simulink model "Test"  (R2018b)
settings: Solver=VariableStepAuto  StartTime=0.0  StopTime=3.0  RelTol=1e-3
libraries: dspvision x6, dspstat3 x5
settings Model: Creator=dell  LastModifiedBy=dell

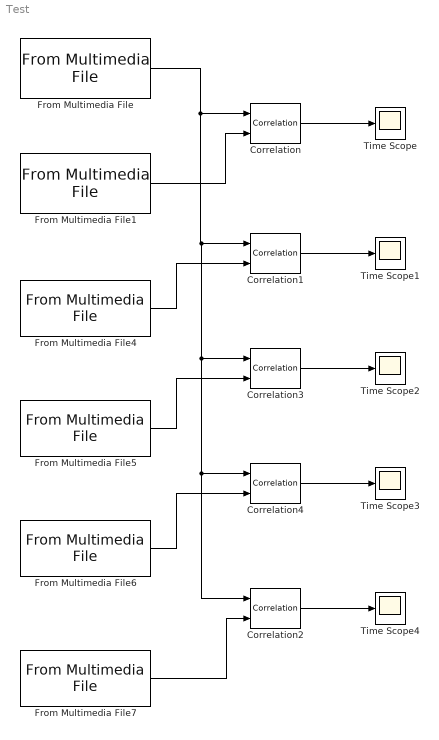
== system Test ==
  Correlation{,1..4} (5 alike) : dspstat3/Correlation  domain=Time  roundingMode=Floor  overflowMode=off  outputDataTypeStr=Inherit: Same as accumulator  outputMin=[]  outputMax=[]  outputLastDataTypeStr=Inherit: Same as accumulator
      settings: SourceProductName=DSP System Toolbox  SourceProductBaseCode=DS
  From Multimedia File : dspvision/From Multimedia File  inputFilename=C:\Users\dell\Desktop\Tone-Identification-master\test.wav  loop=on  numPlays=inf  outputStreams=Audio only  videoDataType=single  audioDataType=double  inheritSampleTime=on  userDefinedSampleTime=1/30  noAudioOutput=off  isIntensityVideo=off  fourcc=RGB  colorVideoFormat=Separate color signals  outputEOF=off  dataOrg=Column-major  audioFrameSize=10000  computeAudioFrameSize=off  outSamplingMode=Sample based
      settings: SourceProductBaseCode=VP
  From Multimedia File1 : dspvision/From Multimedia File  inputFilename=C:\Users\dell\Desktop\Tone-Identification-master\one.wav  loop=on  numPlays=inf  outputStreams=Audio only  videoDataType=single  audioDataType=double  inheritSampleTime=on  userDefinedSampleTime=1/30  noAudioOutput=off  isIntensityVideo=off  fourcc=RGB  colorVideoFormat=Separate color signals  outputEOF=off  dataOrg=Column-major  audioFrameSize=10000  computeAudioFrameSize=off  outSamplingMode=Sample based
      settings: SourceProductBaseCode=VP
  From Multimedia File4 : dspvision/From Multimedia File  inputFilename=C:\Users\dell\Desktop\Tone-Identification-master\two.wav  loop=on  numPlays=inf  outputStreams=Audio only  videoDataType=single  audioDataType=double  inheritSampleTime=on  userDefinedSampleTime=1/30  noAudioOutput=off  isIntensityVideo=off  fourcc=RGB  colorVideoFormat=Separate color signals  outputEOF=off  dataOrg=Column-major  audioFrameSize=10000  computeAudioFrameSize=off  outSamplingMode=Sample based
      settings: SourceProductBaseCode=VP
  From Multimedia File5 : dspvision/From Multimedia File  inputFilename=C:\Users\dell\Desktop\Tone-Identification-master\three.wav  loop=on  numPlays=inf  outputStreams=Audio only  videoDataType=single  audioDataType=double  inheritSampleTime=on  userDefinedSampleTime=1/30  noAudioOutput=off  isIntensityVideo=off  fourcc=RGB  colorVideoFormat=Separate color signals  outputEOF=off  dataOrg=Column-major  audioFrameSize=10000  computeAudioFrameSize=off  outSamplingMode=Sample based
      settings: SourceProductBaseCode=VP
  From Multimedia File6 : dspvision/From Multimedia File  inputFilename=C:\Users\dell\Desktop\Tone-Identification-master\four.wav  loop=on  numPlays=inf  outputStreams=Audio only  videoDataType=single  audioDataType=double  inheritSampleTime=on  userDefinedSampleTime=1/30  noAudioOutput=off  isIntensityVideo=off  fourcc=RGB  colorVideoFormat=Separate color signals  outputEOF=off  dataOrg=Column-major  audioFrameSize=10000  computeAudioFrameSize=off  outSamplingMode=Sample based
      settings: SourceProductBaseCode=VP
  From Multimedia File7 : dspvision/From Multimedia File  inputFilename=C:\Users\dell\Desktop\Tone-Identification-master\five.wav  loop=on  numPlays=inf  outputStreams=Audio only  videoDataType=single  audioDataType=double  inheritSampleTime=on  userDefinedSampleTime=1/30  noAudioOutput=off  isIntensityVideo=off  fourcc=RGB  colorVideoFormat=Separate color signals  outputEOF=off  dataOrg=Column-major  audioFrameSize=10000  computeAudioFrameSize=off  outSamplingMode=Sample based
      settings: SourceProductBaseCode=VP
  Time Scope{,1..4} (5 alike) : Scope
  wires:
  From Multimedia File/1 -> Correlation2/1, Correlation4/1, Correlation3/1, Correlation1/1, Correlation/1
  From Multimedia File1/1 -> Correlation/2
  Correlation/1 -> Time Scope/1
  From Multimedia File4/1 -> Correlation1/2
  From Multimedia File5/1 -> Correlation3/2
  From Multimedia File6/1 -> Correlation4/2
  From Multimedia File7/1 -> Correlation2/2
  Correlation1/1 -> Time Scope1/1
  Correlation3/1 -> Time Scope2/1
  Correlation4/1 -> Time Scope3/1
  Correlation2/1 -> Time Scope4/1
